simulink subsystem "dynamics"  (R2020a)
settings: Solver=VariableStepAuto  StartTime=0.0  StopTime=10.0  RelTol=1e-3
values from neighbouring files (symbols this model uses):
  initial_altitude = 1373    [configure_simulation.m]    (also in test_kalman.m = 20000)
  initial_velocity = 0    [configure_simulation.m]    (also in test_kalman.m = 5)
  M = molar_mass(gas_species)    [calculate_required_gas.m]    (also in configure_simulation.m = molar_mass(lift_gas); evaluate_accel.m; evaluate_jacobian.m; gas_for_equilibrium.m)
settings Model: Creator=Philip  LastModifiedBy=Philip

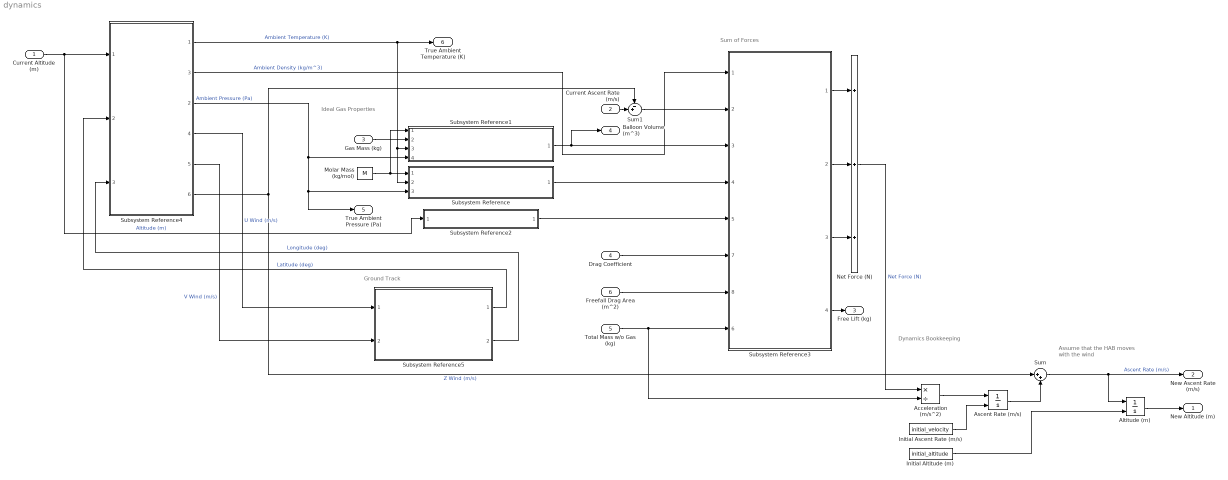
== system dynamics ==
  note: Ground Track
  note: Assume that the HAB moves with the wind
  note: Dynamics Bookkeeping
  note: Sum of Forces
  note: Ideal Gas Properties
  Current Altitude (m) : Inport
  Current Ascent Rate (m/s) : Inport  Port=2
  Gas Mass (kg) : Inport  Port=3
  Drag Coefficient : Inport  Port=4
  Total Mass w/o Gas (kg) : Inport  Port=5
  Freefall Drag Area (m^2) : Inport  Port=6
  Acceleration (m/s^2) : Product  Inputs=*/
  Altitude (m) : Integrator  InitialConditionSource=external
  Ascent Rate (m/s) : Integrator  InitialConditionSource=external
  Initial Altitude (m) : Constant  Value=initial_altitude
  Initial Ascent Rate (m/s) : Constant  Value=initial_velocity
  Molar Mass (kg/mol) : Constant  Value=M
  Net Force (N) : Sum  Inputs=+++
  Subsystem Reference : Subsystem  ReferencedSubsystem=rho_ideal
  Subsystem Reference1 : Subsystem  ReferencedSubsystem=V_ideal
  Subsystem Reference2 : Subsystem  ReferencedSubsystem=gravity_simple
  Subsystem Reference3 : Subsystem  ReferencedSubsystem=forces
      settings: PortSchema="{\"entries\":[{\"content\":{\"sides\":[{\"content\":{\"connectorIds\":[\"In1\",\"In2\",\"In3\",\"In4\",\"In5\",\"In7\",\"In8\",\"In6\"]},\"type\":\"ConnectorPlacement.EquallySpacedRectSide\",\"uuid\":\"8bbb0a20-6e3b-485b-aaea-741c692b9dea\"},{\"content\":{\"connectorIds\":[\"Out1\",\"Out2\",\"Out3\",\"Out4\"],\"side\":\"RIGHT\"},\"type\":\"ConnectorPlacement.EquallySpacedRectSide\",\"uuid\":\"dcca8bff-3b09-4be9-82b0-6eae043772da\"},{\"content\":{\"connectorIds\":[],\"side\":\"TOP\"},\"type\":\"ConnectorPlacement.EquallySpacedRectSide\",\"uuid\":\"133d7d7b-6bad-4b45-8650-ccc27548d600\"}]},\"type\":\"ConnectorPlacement.EquallySpacedConnector\",\"uuid\":\"8c322394-d67a-48c1-9d65-8d16eb5635ba\"}],\"packageUris\":[\"http://schema.mathworks.com/mf0/Connector/19700101\"],\"version\":\"1.0\"}"
  Subsystem Reference4 : Subsystem  ReferencedSubsystem=atmosphere
      settings: PortSchema="{\"entries\":[{\"content\":{\"sides\":[{\"content\":{\"connectorIds\":[\"In1\",\"In2\",\"In3\"]},\"type\":\"ConnectorPlacement.EquallySpacedRectSide\",\"uuid\":\"c2bdcce4-6c89-4bb0-8d0a-01be451eb4c9\"},{\"content\":{\"connectorIds\":[\"Out1\",\"Out3\",\"Out2\",\"Out4\",\"Out5\",\"Out6\"],\"side\":\"RIGHT\"},\"type\":\"ConnectorPlacement.EquallySpacedRectSide\",\"uuid\":\"e5954c8d-771b-418e-bc55-4e8311742813\"},{\"content\":{\"connectorIds\":[],\"side\":\"TOP\"},\"type\":\"ConnectorPlacement.EquallySpacedRectSide\",\"uuid\":\"711b9516-8293-4a51-98c6-f8b19bfe5767\"}]},\"type\":\"ConnectorPlacement.EquallySpacedConnector\",\"uuid\":\"9f8a9f7d-3a0a-48aa-b956-ad016c94175c\"}],\"packageUris\":[\"http://schema.mathworks.com/mf0/Connector/19700101\"],\"version\":\"1.0\"}"
  Subsystem Reference5 : Subsystem  ReferencedSubsystem=flight_path
  Sum : Sum  Inputs=|++
  Sum1 : Sum  Inputs=-+|
  New Altitude (m) : Outport
  New Ascent Rate (m/s) : Outport  Port=2
  Free Lift (kg) : Outport  Port=3
  Balloon Volume (m^3) : Outport  Port=4
  True Ambient Pressure (Pa) : Outport  Port=5
  True Ambient Temperature (K) : Outport  Port=6
  wires:
  Molar Mass (kg/mol)/1 -> Subsystem Reference/1, Subsystem Reference1/1
  Ascent Rate (m/s)/1 -> Sum/2
  Subsystem Reference3/2 -> Net Force (N)/2
  Current Altitude (m)/1 -> Subsystem Reference4/1, Subsystem Reference2/1  "Altitude (m)"
  Net Force (N)/1 -> Acceleration (m/s^2)/1  "Net Force (N)"
  Acceleration (m/s^2)/1 -> Ascent Rate (m/s)/1
  Subsystem Reference3/1 -> Net Force (N)/1
  Subsystem Reference3/3 -> Net Force (N)/3
  Subsystem Reference2/1 -> Subsystem Reference3/5
  Gas Mass (kg)/1 -> Subsystem Reference1/2
  Current Ascent Rate (m/s)/1 -> Sum1/2
  Altitude (m)/1 -> New Altitude (m)/1
  Subsystem Reference3/4 -> Free Lift (kg)/1
  Total Mass w/o Gas (kg)/1 -> Acceleration (m/s^2)/2, Subsystem Reference3/6
  Initial Ascent Rate (m/s)/1 -> Ascent Rate (m/s)/2
  Initial Altitude (m)/1 -> Altitude (m)/2
  Subsystem Reference1/1 -> Balloon Volume (m^3)/1, Subsystem Reference3/3
  Subsystem Reference/1 -> Subsystem Reference3/4
  Drag Coefficient/1 -> Subsystem Reference3/7
  Freefall Drag Area (m^2)/1 -> Subsystem Reference3/8
  Subsystem Reference4/1 -> True Ambient Temperature (K)/1, Subsystem Reference1/3, Subsystem Reference/2  "Ambient Temperature (K)"
  Subsystem Reference4/3 -> Subsystem Reference3/1  "Ambient Density (kg/m^3)"
  Subsystem Reference4/2 -> Subsystem Reference1/4, True Ambient Pressure (Pa)/1, Subsystem Reference/3  "Ambient Pressure (Pa)"
  Subsystem Reference5/2 -> Subsystem Reference4/3  "Longitude (deg)"
  Subsystem Reference5/1 -> Subsystem Reference4/2  "Latitude (deg)"
  Sum/1 -> New Ascent Rate (m/s)/1, Altitude (m)/1  "Ascent Rate (m/s)"
  Subsystem Reference4/6 -> Sum/1, Sum1/1  "Z Wind (m/s)"
  Subsystem Reference4/4 -> Subsystem Reference5/1  "U Wind (m/s)"
  Subsystem Reference4/5 -> Subsystem Reference5/2  "V Wind (m/s)"
  Sum1/1 -> Subsystem Reference3/2
